simulink library "linear_double_integrator_observer_ccaller"  (R2025b)
settings: Solver=VariableStepAuto  StartTime=0.0  StopTime=10.0  RelTol=1e-3
undefined symbols (not defined in the file): kv, kx, ts_afe
settings Model: Creator=dbagn  LastModifiedBy=dbagn
settings SFSimCC: SimCustomHeaderCode=|
  | #include "linear_double_integrator_observer_simulink.h"
  | #include "linear_double_integrator_observer.h"
settings SFSimCC: SimUserSources=|
  | "linear_double_integrator_observer_simulink.c"
  | "linear_double_integrator_observer.c"
settings SFSimCC: SimUserIncludeDirs=|
  | include
  | src

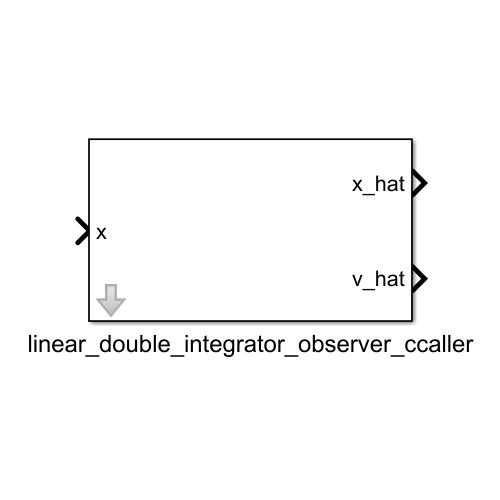
[thumbnail: Simulink's stored preview of the top-level diagram]
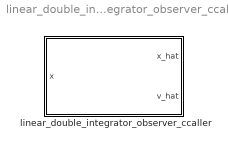
== system linear_double_integrator_observer_ccaller ==
  linear_double_integrator_observer_ccaller : Subsystem  mask{kx_m=kx, kv_m=kv, ts_m=ts_afe, time_release=0.05, instance=0, tc_m=ts_afe}
      mask prompts: kx_m "kx"; kv_m "kv"; ts_m "Sampling Time [s]"; time_release "Reset Time Release [s]"; instance "Instance [#]"; tc_m "Sample Time [s] (-1 for inherited)"

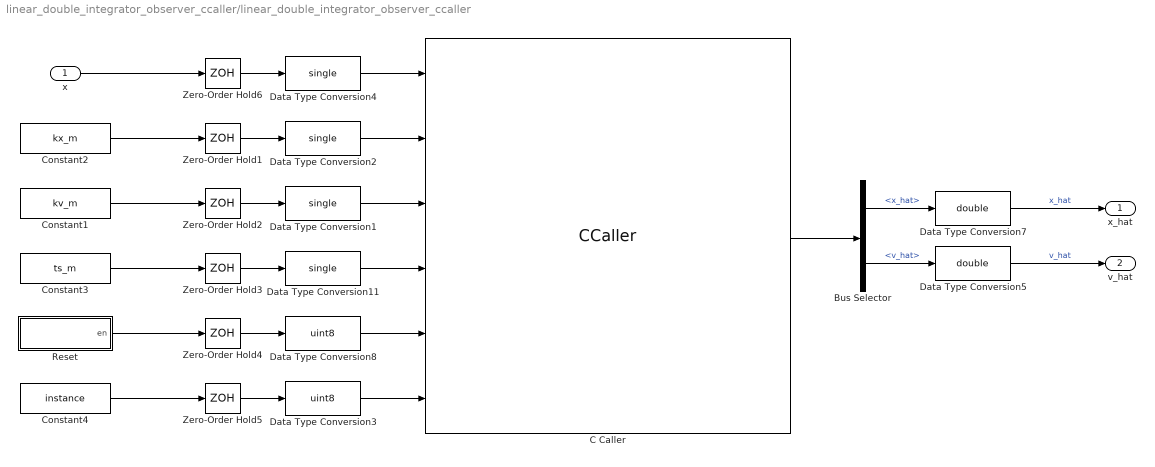
== system linear_double_integrator_observer_ccaller/linear_double_integrator_observer_ccaller ==
  x : Inport
  Bus Selector : BusSelector  OutputSignals=x_hat,v_hat
  C Caller : CCaller  FunctionName=linear_double_integrator_observer_process_simulink  PortSpecificationStruct="%)30     .    , P   8    (     @         %    \"     <    !     0         %  0 \"0    $    _    07)G3F%M90  4&]R=$YA;64 4V-O<&4     26YD97@     5'EP90      4VEZ90      27-';&]B86P   X    P    !@    @    $          4    (     0    ,    !         !   P!O=70 #@   #     &    \"     0         !0    @    !     P    $         $  # &]U=  .    .     8    (    !          %    \"     $    &     0         0   ...(+3831 chars)"  SampleTime=tc_m
  Constant1 : Constant  Value=kv_m
  Constant2 : Constant  Value=kx_m
  Constant3 : Constant  Value=ts_m
  Constant4 : Constant  Value=instance
  Data Type Conversion{1..2,4,11} (4 alike) : DataTypeConversion  OutDataTypeStr=single  SaturateOnIntegerOverflow=off  RndMeth=Floor
  Data Type Conversion3 : DataTypeConversion  OutDataTypeStr=uint8  SaturateOnIntegerOverflow=off  RndMeth=Floor
  Data Type Conversion5 : DataTypeConversion  OutDataTypeStr=double  SaturateOnIntegerOverflow=off  RndMeth=Floor
  Data Type Conversion7 : DataTypeConversion  OutDataTypeStr=double  SaturateOnIntegerOverflow=off  RndMeth=Floor
  Data Type Conversion8 : DataTypeConversion  OutDataTypeStr=uint8  SaturateOnIntegerOverflow=off  RndMeth=Floor
  Reset : Subsystem
  Zero-Order Hold{1..6} (6 alike) : ZeroOrderHold  SampleTime=tc_m
  x_hat : Outport
  v_hat : Outport  Port=2
  wires:
  Bus Selector/2 -> Data Type Conversion5/1  "<v_hat>"
  Data Type Conversion5/1 -> v_hat/1  "v_hat"
  Data Type Conversion7/1 -> x_hat/1  "x_hat"
  C Caller/1 -> Bus Selector/1
  Bus Selector/1 -> Data Type Conversion7/1  "<x_hat>"
  Zero-Order Hold5/1 -> Data Type Conversion3/1
  Data Type Conversion1/1 -> C Caller/3
  Constant1/1 -> Zero-Order Hold2/1
  Data Type Conversion3/1 -> C Caller/6
  Zero-Order Hold1/1 -> Data Type Conversion2/1
  Data Type Conversion11/1 -> C Caller/4
  Zero-Order Hold4/1 -> Data Type Conversion8/1
  Data Type Conversion2/1 -> C Caller/2
  Reset/1(en) -> Zero-Order Hold4/1
  Constant3/1 -> Zero-Order Hold3/1
  Zero-Order Hold2/1 -> Data Type Conversion1/1
  Constant2/1 -> Zero-Order Hold1/1
  Data Type Conversion4/1 -> C Caller/1
  Zero-Order Hold3/1 -> Data Type Conversion11/1
  Data Type Conversion8/1 -> C Caller/5
  Constant4/1 -> Zero-Order Hold5/1
  x/1 -> Zero-Order Hold6/1
  Zero-Order Hold6/1 -> Data Type Conversion4/1

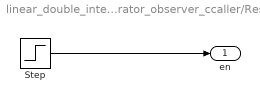
== system linear_double_integrator_observer_ccaller/linear_double_integrator_observer_ccaller/Reset ==
  Step : Step  Time=time_release  Before=1  After=0
  en : Outport
  wires:
  Step/1 -> en/1
